simulink model "pendulum_model"  (R2020a)
settings: Solver=VariableStepAuto  StartTime=0.0  StopTime=10.0  RelTol=1e-3
undefined symbols (not defined in the file): c, g, l, m
settings Model: Creator=Valentina  LastModifiedBy=giaco

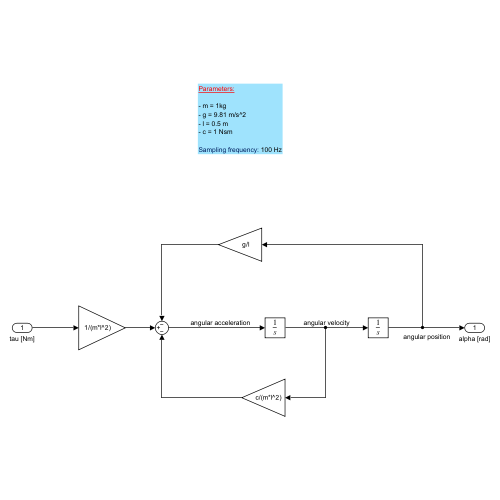
[thumbnail: Simulink's stored preview of the top-level diagram]
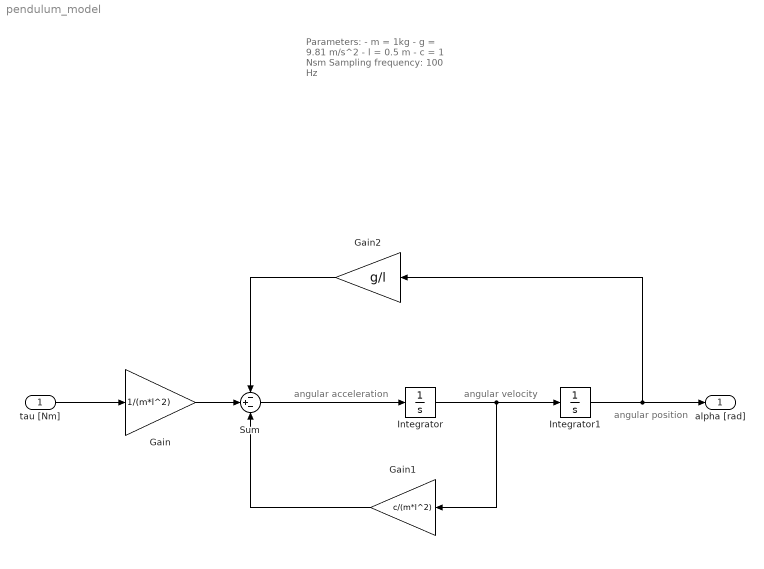
== system pendulum_model ==
  note: Parameters:
      |
      | - m = 1kg
      | - g = 9.81 m/s^2
      | - l = 0.5 m
      | - c = 1 Nsm
      |
      | Sampling frequency: 100 Hz
  note: angular position
  note: angular acceleration
  note: angular velocity
  tau [Nm] : Inport
  Gain : Gain  Gain=1/(m*l^2)
  Gain1 : Gain  Gain=c/(m*l^2)
  Gain2 : Gain  Gain=g/l
  Integrator : Integrator
  Integrator1 : Integrator
  Sum : Sum  Inputs=-+-
  alpha [rad] : Outport
  wires:
  tau [Nm]/1 -> Gain/1
  Gain/1 -> Sum/2
  Sum/1 -> Integrator/1
  Integrator/1 -> Gain1/1, Integrator1/1
  Gain2/1 -> Sum/1
  Gain1/1 -> Sum/3
  Integrator1/1 -> Gain2/1, alpha [rad]/1
